simulink model "mono_kanal"  (R2024a)
settings: Solver=VariableStepAuto  StartTime=0.0  StopTime=1122.0  RelTol=1e-5  AbsTol=1e-6
libraries: simulink x13, matrix_library x3, sharedutil x2, aerolibutil x1
settings Model: Creator=evgenijkondratev  LastModifiedBy=evgenijkondratev

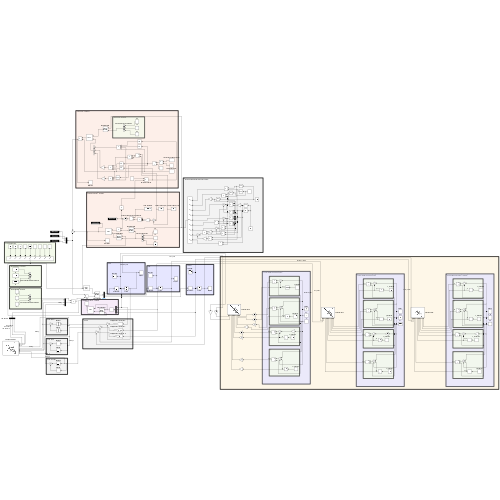
[thumbnail: Simulink's stored preview of the top-level diagram]
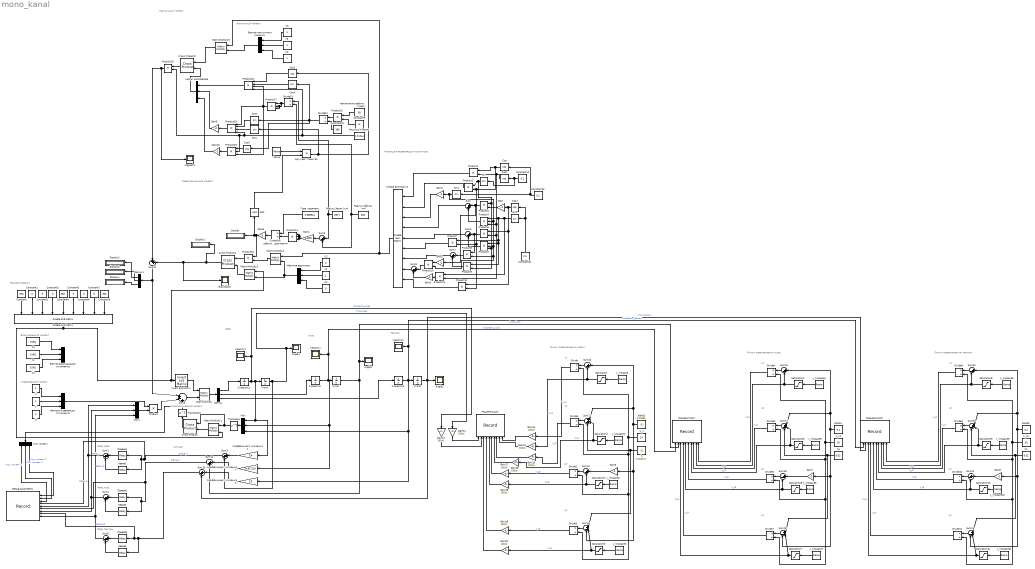
== system mono_kanal ==
  note: L3
  note: L2
  note: Тангаж
  note: L3
  note: L1
  note: Линии переключения (тангаж)
  note: L4
  note: L1
  note: Линии переключения (курс)
  note: Магнитный момент
  note: Реле, курс
  note: L4
  note: L3
  note: L4
  note: Сигнал
  note: L2
  note: Тензор инерции
  note: L2
  note: Реле, тангаж
  note: Магнитный момент
  note: Возмущающий момент
  note: Управляющий момент
  note: Крен
  note: Курс
  note: Реле, крен
  note: Матрица направляющих косинусов
  note: Гироскопический момент
  note: Гравитационный момент
  note: L1
  note: Линии переключения (крен)
  AngleX : Scope
  AngleY : Scope
  AngleZ : Scope
  Constant : Constant  Value=200
  Constant{1..3,5..7} (6 alike) : Constant  Value=0
  Constant10 : Constant  Value=180
  Constant11 : Constant  Value=0.1
  Constant12 : Constant  Value=0.1
  Constant13 : Constant  Value=0.1
  Constant4 : Constant  Value=250
  Constant8 : Constant  Value=300
  Constant9 : Constant  Value=pi
  Cos{,1..3,5} (5 alike) : Trigonometry  Operator=cos
  Cos4 : Trigonometry
  Create 3x3 Matrix : sharedutil/Create 3x3 Matrix  aMode=aMode
      settings: LibrarySourceBlock=aerolibutil/Create 3x3 Matrix
  Create 3x3 Matrix1 : sharedutil/Create 3x3 Matrix  aMode=aMode
      settings: LibrarySourceBlock=aerolibutil/Create 3x3 Matrix
  Cross Product : matrix_library/Cross Product
  Cross Product1 : matrix_library/Cross Product
  Cross Product2 : matrix_library/Cross Product
  Debug parameters : Record  FileSettingsInternal="{\"entries\":[{\"content\":{\"excelSettings\":{\"content\":{},\"type\":\"Streamout.ExcelSettings\"}},\"type\":\"Streamout.FileSettingStorage\",\"uuid\":\"\"}],\"packageUris\":[\"http:\\/\\/schema.mathworks.com\\/mf0\\/streamout_blocks\\/R2020a\"],\"version\":\"1.0\"}"  Layout=[1 1]  SignalsInternal="{\"entries\":[{\"content\":{\"signals\":[{\"content\":{\"blockPath\":[],\"dimensions\":[1,1],\"domain\":\"\",\"lineColor\":\"#a2142f\",\"plots\":[ 1 ],\"port\":1,\"sid\":[\"\"],\"signalID\":1,\"signalName\":\"Гир. момент Z\"},\"type\":\"RecordBlkView.Signal\",\"uuid\":\"\"},{\"content\":{\"blockPath\":[],\"dimensions\":[1,1],\"domain\":\"\",\"lineColor\":\"#139fff\",\"plots\":[ 1 ],\"port\":2,\"sid\":[\"\"],\"signalID\":2,\"signalName\":\"Гир. момент Y\"},\"type\":\"RecordBlkView.Signal\",\"uuid\":\"\"},{\"content\":{\"blockPath\":[],\"dimensions\":[1,1],\"domain\":\"\",\"lineColor\":\"#64d413\",\"lineWidth\":2,\"port\":3,\"sid\":[\"\"],\"signalID\":3,\"signalName\":\"Гир. момент X\"},\"type\":\"RecordBlkView.Signal\",\"uuid\":\"\"},{\"content\":{\"blockPath\":[],\"dimensions\":[1],\"domain\":\"\",\"lineColor\":\"#ff13a6\",\"lineWidth\":2,\"port\":4,\"sid\":[\"\"],\"signalID\":4,\"signalName\":\"Sigma_X\"},\"type\":\"RecordBlkView.Signal\",\"uuid\":\"\"},{\"content\":{\"blockPath\":[],\"dimensions\":[1],\"domain\":\"\",\"lineColor\":\"#fe330a\",\"lineWidth\":2,\"port\":5,\"sid\":[\"\"],\"signalID\":5,\"signalName\":\"Relay_X\"},\"type\":\"RecordBlkView.Signal\",\"uuid\":\"\"},{\"content\":{\"blockPath\":[],\"dimensions\":[1],\"domain\":\"\",\"lineColor\":\"#22b573\",\"lineWidth\":2,\"port\":6,\"sid\":[\"\"],\"signalID\":6,\"signalName\":\"Sigma_Y\"},\"type\":\"RecordBlkView.Signal\",\"uuid\":\"\"},{\"content\":{\"blockPath\":[],\"dimensions\":[1],\"domain\":\"\",\"lineColor\":\"#0072bd\",\"lineWidth\":2,\"port\":7,\"sid\":[\"\"],\"signalID\":7,\"signalName\":\"Relay_Y\"},\"type\":\"RecordBlkView.Signal\",\"uuid\":\"\"},{\"content\":{\"blockPath\":[],\"dimensions\":[1],\"domain\":\"\",\"lineColor\":\"#d95319\",\"lineWidth\":2,\"port\":8,\"sid\":[\"\"],\"signalID\":8,\"signalName\":\"Sigma_Z\"},\"type\":\"RecordBlkView.Signal\",\"uuid\":\"\"},{\"content\":{\"blockPath\":[],\"dimensions\":[1],\"domain\":\"\",\"lineColor\":\"#edb120\",\"lineWidth\":2,\"port\":9,\"sid\":[\"\"],\"signalID\":9,\"signalName\":\"Relay_Z\"},\"type\":\"RecordBlkView.Signal\",\"uuid\":\"\"}]},\"type\":\"RecordBlkView.InputSignals\",\"uuid\":\"\"}],\"packageUris\":[\"http:\\/\\/schema.mathworks.com\\/mf0\\/streamout_blocks\\/R2020a\"],\"version\":\"1.0\"}"  VisualizationBindings="{\"xyplotplugin\":{\"info\":[{\"series\":[{\"bindingParametersList\":[{\"parameter\":\"X-Axis\",\"signalID\":1,\"signalName\":\"Гир. момент Z\"},{\"parameter\":\"Y-Axis\",\"signalID\":2,\"signalName\":\"Гир. момент Y\"}],\"seriesID\":0}],\"subplotID\":1}]}}"  CompatibilityTag=XY
  Demux : Demux  Outputs=3
  Demux1 : Demux  Outputs=3
  Display{,1..4} (5 alike) : Display
  Divide{,1..13} (14 alike) : Product  Inputs=*/
  Gain{,1..3,6..8,10} (8 alike) : Gain  Gain=-1
  Gain{11..20} (10 alike) : Gain  Gain=180/pi
  Gain4 : Gain  Gain=1000
  Gain5 : Gain  Gain=3
  Gain9 : Gain  Gain=-2
  Gravitation : Scope
  Invert 3x3 Matrix : aerolibutil/Invert  3x3 Matrix
  Magnetic : Scope
  MatrixMultiply{,1..3,5} (5 alike) : Product  Multiplication=Matrix(*)
  Mux : Mux  Inputs=3
  Mux1 : Mux  Inputs=3
  PhasePortraitX : Record  FileSettingsInternal="{\"entries\":[{\"content\":{\"excelSettings\":{\"content\":{},\"type\":\"Streamout.ExcelSettings\"}},\"type\":\"Streamout.FileSettingStorage\",\"uuid\":\"\"}],\"packageUris\":[\"http:\\/\\/schema.mathworks.com\\/mf0\\/streamout_blocks\\/R2020a\"],\"version\":\"1.0\"}"  Layout=[1 1]  SignalsInternal="{\"entries\":[{\"content\":{\"signals\":[{\"content\":{\"blockPath\":[],\"dimensions\":[1],\"domain\":\"\",\"lineColor\":\"#a2142f\",\"lineWidth\":2,\"port\":1,\"sid\":[\"\"],\"signalID\":1,\"signalName\":\"Gain11\"},\"type\":\"RecordBlkView.Signal\",\"uuid\":\"\"},{\"content\":{\"blockPath\":[],\"dimensions\":[1],\"domain\":\"\",\"lineColor\":\"#139fff\",\"lineWidth\":2,\"port\":2,\"sid\":[\"\"],\"signalID\":2,\"signalName\":\"Gain12\"},\"type\":\"RecordBlkView.Signal\",\"uuid\":\"\"},{\"content\":{\"blockPath\":[],\"dimensions\":[1],\"domain\":\"\",\"lineColor\":\"#ff6929\",\"lineWidth\":2,\"port\":3,\"sid\":[\"\"],\"signalID\":3,\"signalName\":\"Gain20\"},\"type\":\"RecordBlkView.Signal\",\"uuid\":\"\"},{\"content\":{\"blockPath\":[],\"dimensions\":[1],\"domain\":\"\",\"lineColor\":\"#b746ff\",\"lineWidth\":2,\"port\":4,\"sid\":[\"\"],\"signalID\":4,\"signalName\":\"Gain19\"},\"type\":\"RecordBlkView.Signal\",\"uuid\":\"\"},{\"content\":{\"blockPath\":[],\"dimensions\":[1],\"domain\":\"\",\"lineColor\":\"#64d413\",\"lineWidth\":2,\"port\":5,\"sid\":[\"\"],\"signalID\":5,\"signalName\":\"Gain18\"},\"type\":\"RecordBlkView.Signal\",\"uuid\":\"\"},{\"content\":{\"blockPath\":[],\"dimensions\":[1],\"domain\":\"\",\"lineColor\":\"#ff13a6\",\"lineWidth\":2,\"port\":6,\"sid\":[\"\"],\"signalID\":6,\"signalName\":\"Gain17\"},\"type\":\"RecordBlkView.Signal\",\"uuid\":\"\"},{\"content\":{\"blockPath\":[],\"dimensions\":[1],\"domain\":\"\",\"lineColor\":\"#fe330a\",\"lineWidth\":2,\"port\":7,\"sid\":[\"\"],\"signalID\":7,\"signalName\":\"Gain16\"},\"type\":\"RecordBlkView.Signal\",\"uuid\":\"\"},{\"content\":{\"blockPath\":[],\"dimensions\":[1],\"domain\":\"\",\"lineColor\":\"#22b573\",\"lineWidth\":2,\"port\":8,\"sid\":[\"\"],\"signalID\":8,\"signalName\":\"Gain15\"},\"type\":\"RecordBlkView.Signal\",\"uuid\":\"\"},{\"content\":{\"blockPath\":[],\"dimensions\":[1],\"domain\":\"\",\"lineColor\":\"#0072bd\",\"lineWidth\":2,\"port\":9,\"sid\":[\"\"],\"signalID\":9,\"signalName\":\"Gain14\"},\"type\":\"RecordBlkView.Signal\",\"uuid\":\"\"},{\"content\":{\"blockPath\":[],\"dimensions\":[1],\"domain\":\"\",\"lineColor\":\"#d95319\",\"lineWidth\":2,\"port\":10,\"sid\":[\"\"],\"signalID\":10,\"signalName\":\"Gain13\"},\"type\":\"RecordBlkView.Signal\",\"uuid\":\"\"}]},\"type\":\"RecordBlkView.InputSignals\",\"uuid\":\"\"}],\"packageUris\":[\"http:\\/\\/schema.mathworks.com\\/mf0\\/streamout_blocks\\/R2020a\"],\"version\":\"1.0\"}"  VisualizationBindings="{\"xyplotplugin\":{\"info\":[{\"series\":[],\"subplotID\":1}]}}"  CompatibilityTag=XY
  PhasePortraitY : Record  FileSettingsInternal="{\"entries\":[{\"content\":{\"excelSettings\":{\"content\":{},\"type\":\"Streamout.ExcelSettings\"}},\"type\":\"Streamout.FileSettingStorage\",\"uuid\":\"\"}],\"packageUris\":[\"http:\\/\\/schema.mathworks.com\\/mf0\\/streamout_blocks\\/R2020a\"],\"version\":\"1.0\"}"  Layout=[1 1]  SignalsInternal="{\"entries\":[{\"content\":{\"signals\":[{\"content\":{\"blockPath\":[],\"dimensions\":[1],\"domain\":\"\",\"lineColor\":\"#edb120\",\"lineWidth\":2,\"port\":1,\"sid\":[\"\"],\"signalID\":1,\"signalName\":\"Скорость_курс\"},\"type\":\"RecordBlkView.Signal\",\"uuid\":\"\"},{\"content\":{\"blockPath\":[],\"dimensions\":[1],\"domain\":\"\",\"lineColor\":\"#7e2f8e\",\"lineWidth\":2,\"port\":2,\"sid\":[\"\"],\"signalID\":2,\"signalName\":\"Угол_Курс\"},\"type\":\"RecordBlkView.Signal\",\"uuid\":\"\"},{\"content\":{\"blockPath\":[],\"dimensions\":[1],\"domain\":\"\",\"lineColor\":\"#77ac30\",\"lineWidth\":2,\"port\":3,\"sid\":[\"\"],\"signalID\":3,\"signalName\":\"X_L4\"},\"type\":\"RecordBlkView.Signal\",\"uuid\":\"\"},{\"content\":{\"blockPath\":[],\"dimensions\":[1],\"domain\":\"\",\"lineColor\":\"#4dbeee\",\"lineWidth\":2,\"port\":4,\"sid\":[\"\"],\"signalID\":4,\"signalName\":\"Y_L4\"},\"type\":\"RecordBlkView.Signal\",\"uuid\":\"\"},{\"content\":{\"blockPath\":[],\"dimensions\":[1],\"domain\":\"\",\"lineColor\":\"#a2142f\",\"lineWidth\":2,\"port\":5,\"sid\":[\"\"],\"signalID\":5,\"signalName\":\"X_L3\"},\"type\":\"RecordBlkView.Signal\",\"uuid\":\"\"},{\"content\":{\"blockPath\":[],\"dimensions\":[1],\"domain\":\"\",\"lineColor\":\"#139fff\",\"lineWidth\":2,\"port\":6,\"sid\":[\"\"],\"signalID\":6,\"signalName\":\"Y_L3\"},\"type\":\"RecordBlkView.Signal\",\"uuid\":\"\"},{\"content\":{\"blockPath\":[],\"dimensions\":[1],\"domain\":\"\",\"lineColor\":\"#ff6929\",\"lineWidth\":2,\"port\":7,\"sid\":[\"\"],\"signalID\":7,\"signalName\":\"X_L2\"},\"type\":\"RecordBlkView.Signal\",\"uuid\":\"\"},{\"content\":{\"blockPath\":[],\"dimensions\":[1],\"domain\":\"\",\"lineColor\":\"#b746ff\",\"lineWidth\":2,\"port\":8,\"sid\":[\"\"],\"signalID\":8,\"signalName\":\"Y_L2\"},\"type\":\"RecordBlkView.Signal\",\"uuid\":\"\"},{\"content\":{\"blockPath\":[],\"dimensions\":[1],\"domain\":\"\",\"lineColor\":\"#64d413\",\"lineWidth\":2,\"port\":9,\"sid\":[\"\"],\"signalID\":9,\"signalName\":\"X_L1\"},\"type\":\"RecordBlkView.Signal\",\"uuid\":\"\"},{\"content\":{\"blockPath\":[],\"dimensions\":[1],\"domain\":\"\",\"lineColor\":\"#ff13a6\",\"lineWidth\":2,\"port\":10,\"sid\":[\"\"],\"signalID\":10,\"signalName\":\"Y_L1\"},\"type\":\"RecordBlkView.Signal\",\"uuid\":\"\"}]},\"type\":\"RecordBlkView.InputSignals\",\"uuid\":\"\"}],\"packageUris\":[\"http:\\/\\/schema.mathworks.com\\/mf0\\/streamout_blocks\\/R2020a\"],\"version\":\"1.0\"}"  VisualizationBindings="{\"xyplotplugin\":{\"info\":[{\"series\":[],\"subplotID\":1}]}}"  CompatibilityTag=XY
  PhasePortraitZ : Record  FileSettingsInternal="{\"entries\":[{\"content\":{\"excelSettings\":{\"content\":{},\"type\":\"Streamout.ExcelSettings\"}},\"type\":\"Streamout.FileSettingStorage\",\"uuid\":\"\"}],\"packageUris\":[\"http:\\/\\/schema.mathworks.com\\/mf0\\/streamout_blocks\\/R2020a\"],\"version\":\"1.0\"}"  Layout=[1 1]  SignalsInternal="{\"entries\":[{\"content\":{\"signals\":[{\"content\":{\"blockPath\":[],\"dimensions\":[1],\"domain\":\"\",\"lineColor\":\"#fe330a\",\"plots\":[ 1 ],\"port\":1,\"sid\":[\"\"],\"signalID\":1,\"signalName\":\"Скорость_тангаж\"},\"type\":\"RecordBlkView.Signal\",\"uuid\":\"\"},{\"content\":{\"blockPath\":[],\"dimensions\":[1],\"domain\":\"\",\"lineColor\":\"#139fff\",\"plots\":[ 1 ],\"port\":2,\"sid\":[\"\"],\"signalID\":2,\"signalName\":\"Угол_тангаж\"},\"type\":\"RecordBlkView.Signal\",\"uuid\":\"\"},{\"content\":{\"blockPath\":[],\"dimensions\":[1],\"domain\":\"\",\"lineColor\":\"#fe330a\",\"lineWidth\":2,\"port\":3,\"sid\":[\"\"],\"signalID\":3,\"signalName\":\"X_L4\"},\"type\":\"RecordBlkView.Signal\",\"uuid\":\"\"},{\"content\":{\"blockPath\":[],\"dimensions\":[1],\"domain\":\"\",\"lineColor\":\"#22b573\",\"lineWidth\":2,\"port\":4,\"sid\":[\"\"],\"signalID\":4,\"signalName\":\"Y_L4\"},\"type\":\"RecordBlkView.Signal\",\"uuid\":\"\"},{\"content\":{\"blockPath\":[],\"dimensions\":[1],\"domain\":\"\",\"lineColor\":\"#0072bd\",\"lineWidth\":2,\"port\":5,\"sid\":[\"\"],\"signalID\":5,\"signalName\":\"X_L3\"},\"type\":\"RecordBlkView.Signal\",\"uuid\":\"\"},{\"content\":{\"blockPath\":[],\"dimensions\":[1],\"domain\":\"\",\"lineColor\":\"#d95319\",\"lineWidth\":2,\"port\":6,\"sid\":[\"\"],\"signalID\":6,\"signalName\":\"Y_L3\"},\"type\":\"RecordBlkView.Signal\",\"uuid\":\"\"},{\"content\":{\"blockPath\":[],\"dimensions\":[1],\"domain\":\"\",\"lineColor\":\"#edb120\",\"lineWidth\":2,\"port\":7,\"sid\":[\"\"],\"signalID\":7,\"signalName\":\"X_L2\"},\"type\":\"RecordBlkView.Signal\",\"uuid\":\"\"},{\"content\":{\"blockPath\":[],\"dimensions\":[1],\"domain\":\"\",\"lineColor\":\"#7e2f8e\",\"lineWidth\":2,\"port\":8,\"sid\":[\"\"],\"signalID\":8,\"signalName\":\"Y_L2\"},\"type\":\"RecordBlkView.Signal\",\"uuid\":\"\"},{\"content\":{\"blockPath\":[],\"dimensions\":[1],\"domain\":\"\",\"lineColor\":\"#77ac30\",\"lineWidth\":2,\"port\":9,\"sid\":[\"\"],\"signalID\":9,\"signalName\":\"X_L1\"},\"type\":\"RecordBlkView.Signal\",\"uuid\":\"\"},{\"content\":{\"blockPath\":[],\"dimensions\":[1],\"domain\":\"\",\"lineColor\":\"#4dbeee\",\"lineWidth\":2,\"port\":10,\"sid\":[\"\"],\"signalID\":10,\"signalName\":\"Y_L1\"},\"type\":\"RecordBlkView.Signal\",\"uuid\":\"\"}]},\"type\":\"RecordBlkView.InputSignals\",\"uuid\":\"\"}],\"packageUris\":[\"http:\\/\\/schema.mathworks.com\\/mf0\\/streamout_blocks\\/R2020a\"],\"version\":\"1.0\"}"  VisualizationBindings="{\"xyplotplugin\":{\"info\":[{\"series\":[{\"bindingParametersList\":[{\"parameter\":\"X-Axis\",\"signalID\":1,\"signalName\":\"Скорость_тангаж\"},{\"parameter\":\"Y-Axis\",\"signalID\":2,\"signalName\":\"Угол_тангаж\"}],\"seriesID\":0}],\"subplotID\":1}]}}"  CompatibilityTag=XY
  Product{,1..3,5,7..13,15,20} (14 alike) : Product
  Product{4,6,14,17,19} (5 alike) : Product  Inputs=3
  Product16 : Product  Inputs=4
  Product18 : Product  Inputs=4
  Ramp : simulink/Sources/Ramp  slope=1  start=0  InitialOutput=0
  Saturation{,1..11} (12 alike) : Saturate  UpperLimit=0.15  LowerLimit=-0.15
  Sin{,1..4} (5 alike) : Trigonometry
  Sqrt : Sqrt
  Sum{,1,3..9,14..15,24} (12 alike) : Sum  Inputs=|++
  Sum{10,12,16,18,20,22} (6 alike) : Sum  Inputs=|+-
  Sum{11,13,17,19,21,23} (6 alike) : Sum  Inputs=|+--
  Sum2 : Sum  Inputs=|+-+
  Transpose : Math  Operator=transpose
  Transpose1 : Math  Operator=transpose
  Vector Concatenate : Concatenate  NumInputs=3
  VelocityX : Scope
  VelocityY : Scope
  VelocityZ : Scope
  X : Constant
  X1 : Constant  Value=0.001
  X2 : Constant  Value=0
  X3 : Constant
  Y : Constant
  Y1 : Constant  Value=0.001
  Y2 : Constant
  Y3 : Constant
  Z : Constant
  Z1 : Constant  Value=0.001
  Z2 : Constant  Value=0
  Z3 : Constant
  alpha1 : Constant  Value=0.1
  alpha2 : Constant  Value=0.00698
  alpha3 : Constant  Value=0.1
  h : Constant  Value=0.002617
  h1 : Constant  Value=0.02
  h2 : Constant  Value=0.02
  k_x : Constant  Value=14
  k_x1 : Constant  Value=10
  k_x2 : Constant  Value=10
  x_linspace{,1..11} (12 alike) : simulink/Sources/Ramp  slope=1  start=0  InitialOutput=-1
  Аргумент перигея : Product
  Вектор возмущающего момента : Concatenate  NumInputs=3
  Вектор магнитного момента : Concatenate  NumInputs=3
  Вектор управляющего момента : Concatenate  NumInputs=3
  Гир. момент : Demux  Outputs=3
  Грав. параметр : Constant  Value=3.986e14
  Индукция Земли : Constant  Value=0.315e-4
  Коэффициент усиления X : Gain  Gain=14
  Коэффициент усиления Y : Gain  Gain=14.617224
  Коэффициент усиления Z : Gain  Gain=10
  Левое1 : Relay  OnSwitchValue=-0.00698+0.002617  OffSwitchValue=-0.00698  OnOutputValue=0  OffOutputValue=-1
  Левое2 : Relay  OnSwitchValue=-0.08  OffSwitchValue=-0.1  OnOutputValue=0  OffOutputValue=-1
  Левое3 : Relay  OnSwitchValue=-0.08  OffSwitchValue=-0.1  OnOutputValue=0  OffOutputValue=-1
  Местная вертикаль : Concatenate  NumInputs=3
  Наклонение орбиты (град) : Constant  Value=50
  Правое1 : Relay  OnSwitchValue=0.00698  OffSwitchValue=0.00698-0.002617
  Правое2 : Relay  OnSwitchValue=0.1  OffSwitchValue=0.08
  Правое3 : Relay  OnSwitchValue=0.1  OffSwitchValue=0.08
  Радиус Земли (км) : Constant  Value=6371
  Радиус орбиты (км) : Constant  Value=820
  Скорость орбитального движения : Product  Inputs=*/
  СкоростьX : Integrator  InitialCondition=0.000114843
  СкоростьY : Integrator  InitialCondition=0.001
  СкоростьZ : Integrator  InitialCondition=0.001
  УголX : Integrator  InitialCondition=-0.0017558
  УголY : Integrator  InitialCondition=0.001
  УголZ : Integrator  InitialCondition=0.001
  wires:
  Gain1/1 -> Create 3x3 Matrix1/3
  Product3/1 -> Gain2/1, Sum/1
  Divide3/1 -> Gain19/1  "Y_L4"
  Sum22/1 -> Divide10/1
  Transpose1/1 -> Гир. момент/1
  Vector Concatenate/1 -> Cross Product2/2
  Sum6/1 -> Create 3x3 Matrix1/5
  Sum21/1 -> Divide9/1
  Sum13/1 -> Divide3/1
  Местная вертикаль/1 -> MatrixMultiply3/2, MatrixMultiply2/2
  Saturation4/1 -> PhasePortraitY/9, Sum16/2  "X_L1"
  Радиус орбиты (км)/1 -> Sum9/2, Divide13/2
  x_linspace2/1 -> Saturation2/1
  Sum11/1 -> Divide1/1
  УголY/1 -> PhasePortraitY/2, AngleY/1, Sum14/2  "Угол_Курс"
  x_linspace9/1 -> Saturation9/1
  Product6/1 -> Sum6/2
  X2/1 -> Местная вертикаль/1
  УголZ/1 -> PhasePortraitZ/2, Sum15/2, AngleZ/1  "Угол_тангаж"
  Gain4/1 -> Product14/1, Product14/2, Product14/3
  Gain2/1 -> Product10/1
  x_linspace8/1 -> Saturation8/1
  Sin/1 -> Product2/1, Product9/2, Product6/3, Product3/1
  Gain6/1 -> Sum12/1
  Divide10/1 -> PhasePortraitZ/6  "Y_L3"
  alpha1/1 -> Gain7/1, Sum19/3, Sum17/1, Sum16/1
  Sum15/1 -> Левое3/1, Debug parameters/8, Правое3/1  "Sigma_Z"
  Sum17/1 -> Divide5/1
  x_linspace10/1 -> Saturation10/1
  Z1/1 -> Вектор возмущающего момента/3
  Mux1/1 -> Product/2
  h1/1 -> Sum17/3, Sum19/1
  Product1/1 -> Create 3x3 Matrix1/1
  x_linspace1/1 -> Saturation1/1
  Product19/1 -> Gain10/1
  h2/1 -> Sum21/3, Sum23/1
  Ramp/1 -> Аргумент перигея/1
  Коэффициент усиления Y/1 -> Sum14/1
  Saturation7/1 -> PhasePortraitY/3, Sum19/2  "X_L4"
  Demux/3 -> СкоростьZ/1
  MatrixMultiply1/1 -> Cross Product/2
  Sum18/1 -> Divide6/1
  Sqrt/1 -> Аргумент перигея/2
  Sum12/1 -> Divide2/1
  Product4/1 -> Sum/2
  k_x/1 -> Divide3/2, Divide2/2, Divide1/2, Divide/2
  Sum8/1 -> Create 3x3 Matrix1/8
  Скорость орбитального движения/1 -> Gain5/1
  k_x2/1 -> Divide11/2, Divide10/2, Divide9/2, Divide8/2
  Cos1/1 -> Product1/2, Product11/2, Product5/2, Product4/3
  x_linspace11/1 -> Saturation11/1
  Product12/1 -> Create 3x3 Matrix1/9
  alpha3/1 -> Gain8/1, Sum23/3, Sum21/1, Sum20/1
  Product8/1 -> Sum7/1
  Saturation3/1 -> Gain20/1, Sum13/2  "X_L4"
  k_x1/1 -> Divide7/2, Divide6/2, Divide5/2, Divide4/2
  Вектор управляющего момента/1 -> Product/1
  Divide5/1 -> PhasePortraitY/8  "Y_L2"
  Sum4/1 -> Mux1/2, Debug parameters/7  "Relay_Y"
  Product14/1 -> Скорость орбитального движения/2
  Create 3x3 Matrix1/1 -> MatrixMultiply5/1, MatrixMultiply2/1
  MatrixMultiply5/1 -> Cross Product2/1
  Sum10/1 -> Divide/1
  Transpose/1 -> Cross Product/1, MatrixMultiply1/1
  x_linspace/1 -> Saturation/1
  Gain/1 -> Product3/2
  Create 3x3 Matrix/1 -> MatrixMultiply3/1, Invert 3x3 Matrix/1, MatrixMultiply1/2
  Invert 3x3 Matrix/1 -> MatrixMultiply/1
  MatrixMultiply/1 -> Demux/1
  Грав. параметр/1 -> Скорость орбитального движения/1
  Cross Product1/1 -> Display1/1, Sum24/2, Gravitation/1
  Product10/1 -> Sum8/1
  Sin2/1 -> Product11/1, Product6/1, Product9/1, Product7/1, Product4/1
  Product2/1 -> Create 3x3 Matrix1/2
  Cos3/1 -> Product16/1
  УголX/1 -> Gain11/1, AngleX/1, Sum3/2  "Угол_крен"
  h/1 -> Sum11/3, Sum13/1
  x_linspace7/1 -> Saturation7/1
  Product9/1 -> Sum7/2
  Saturation9/1 -> PhasePortraitZ/7, Sum21/2  "X_L2"
  Sum/1 -> Create 3x3 Matrix1/4
  Saturation2/1 -> Gain18/1, Sum12/2  "X_L3"
  Constant6/1 -> Create 3x3 Matrix/7
  Saturation1/1 -> Gain16/1, Sum11/2  "X_L2"
  Cos2/1 -> Product12/1, Product5/1, Gain/1
  Gain10/1 -> Vector Concatenate/3
  Z/1 -> Вектор управляющего момента/3
  X/1 -> Вектор управляющего момента/1
  Product18/1 -> Gain9/1
  Sum3/1 -> Debug parameters/4, Левое1/1, Правое1/1  "Sigma_X"
  X1/1 -> Вектор возмущающего момента/1
  Constant1/1 -> Create 3x3 Matrix/2
  Constant4/1 -> Create 3x3 Matrix/5
  Constant10/1 -> Divide12/2
  Gain7/1 -> Sum18/1
  Z2/1 -> Местная вертикаль/3
  Constant7/1 -> Create 3x3 Matrix/8
  Sum24/1 -> Sum2/1, Demux1/1
  Y1/1 -> Вектор возмущающего момента/2
  Sum2/1 -> MatrixMultiply/2
  Гир. момент/1 -> Debug parameters/3  "Гир. момент X"
  Product13/1 -> Cross Product1/1
  Product17/1 -> Product19/3, Product18/1, Product16/3
  Наклонение орбиты (град)/1 -> Product15/1
  Левое1/1 -> Sum1/2
  Saturation11/1 -> PhasePortraitZ/3, Sum23/2  "X_L4"
  СкоростьZ/1 -> PhasePortraitZ/1, VelocityZ/1, Коэффициент усиления Z/1, Mux/3, УголZ/1  "Скорость_тангаж"
  Y2/1 -> Местная вертикаль/2
  Правое3/1 -> Sum5/1
  Constant/1 -> Create 3x3 Matrix/1
  Product/1 -> Sum2/2
  Gain3/1 -> Sum8/2
  Sum1/1 -> Mux1/1, Debug parameters/5  "Relay_X"
  Sum5/1 -> Mux1/3, Debug parameters/9  "Relay_Z"
  Sum14/1 -> Левое2/1, Правое2/1, Debug parameters/6  "Sigma_Y"
  Product7/1 -> Create 3x3 Matrix1/6
  Constant2/1 -> Create 3x3 Matrix/3
  Demux/1 -> СкоростьX/1
  Гир. момент/2 -> Debug parameters/2  "Гир. момент Y"
  Cos/1 -> Product1/1, Product12/2, Product7/2, Product2/2
  Правое1/1 -> Sum1/1
  Индукция Земли/1 -> Product20/2, Product19/2, Product18/4, Product16/4
  Gain8/1 -> Sum22/1
  Product11/1 -> Gain3/1
  Product5/1 -> Product8/1, Sum6/1
  Gain9/1 -> Vector Concatenate/2
  x_linspace3/1 -> Saturation3/1
  Saturation6/1 -> PhasePortraitY/5, Sum18/2  "X_L3"
  Sum7/1 -> Create 3x3 Matrix1/7
  Divide9/1 -> PhasePortraitZ/8  "Y_L2"
  СкоростьY/1 -> VelocityY/1, PhasePortraitY/1, Mux/2, Коэффициент усиления Y/1, УголY/1  "Скорость_курс"
  Sin3/1 -> Product18/2
  Saturation/1 -> Gain14/1, Sum10/2  "X_L1"
  Divide6/1 -> PhasePortraitY/6  "Y_L3"
  Constant8/1 -> Create 3x3 Matrix/9
  Cos5/1 -> Product19/1
  Constant5/1 -> Create 3x3 Matrix/6
  Sum9/1 -> Gain4/1
  Sum23/1 -> Divide11/1
  Divide2/1 -> Gain17/1  "Y_L3"
  Cos4/1 -> Product16/2
  Demux/2 -> СкоростьY/1
  Product16/1 -> Vector Concatenate/1
  Divide1/1 -> Gain15/1  "Y_L2"
  Аргумент перигея/1 -> Sin4/1, Cos3/1
  Гир. момент/3 -> Debug parameters/1  "Гир. момент Z"
  Правое2/1 -> Sum4/1
  Gain5/1 -> Display/1, Sqrt/1, Product13/1
  Divide11/1 -> PhasePortraitZ/4  "Y_L4"
  Cross Product/1 -> Transpose1/1
  Y/1 -> Вектор управляющего момента/2
  Радиус Земли (км)/1 -> Divide13/1, Sum9/1
  Constant9/1 -> Product15/2
  Saturation5/1 -> PhasePortraitY/7, Sum17/2  "X_L2"
  alpha2/1 -> Gain6/1, Sum13/3, Sum11/1, Sum10/1
  Saturation8/1 -> PhasePortraitZ/9, Sum20/2  "X_L1"
  Коэффициент усиления X/1 -> Sum3/1
  Y3/1 -> Вектор магнитного момента/2
  Коэффициент усиления Z/1 -> Sum15/1
  x_linspace5/1 -> Saturation5/1
  Product15/1 -> Divide12/1
  Sum16/1 -> Divide4/1
  Divide13/1 -> Product17/1, Product17/3, Product17/2
  x_linspace6/1 -> Saturation6/1
  Z3/1 -> Вектор магнитного момента/3
  x_linspace4/1 -> Saturation4/1
  Sin1/1 -> Product10/2, Product8/2, Product6/2, Product4/2, Gain1/1
  Divide12/1 -> Sin3/1, Cos4/1, Cos5/1
  MatrixMultiply2/1 -> Product13/2
  Sum19/1 -> Divide7/1
  Product20/1 -> Sum24/1, Magnetic/1
  Mux/1 -> Transpose/1
  Divide/1 -> Gain13/1  "Y_L1"
  Saturation10/1 -> PhasePortraitZ/5, Sum22/2  "X_L3"
  Cross Product2/1 -> Product20/1
  Divide8/1 -> PhasePortraitZ/10  "Y_L1"
  Левое2/1 -> Sum4/2
  MatrixMultiply3/1 -> Cross Product1/2
  Divide4/1 -> PhasePortraitY/10  "Y_L1"
  Sin4/1 -> Product18/3
  Divide7/1 -> PhasePortraitY/4  "Y_L4"
  Вектор магнитного момента/1 -> MatrixMultiply5/2
  Sum20/1 -> Divide8/1
  СкоростьX/1 -> VelocityX/1, Gain12/1, Mux/1, Коэффициент усиления X/1, УголX/1  "Скорость_крен"
  X3/1 -> Вектор магнитного момента/1
  Constant3/1 -> Create 3x3 Matrix/4
  Левое3/1 -> Sum5/2
  Constant11/1 -> Sin2/1, Cos2/1
  Constant12/1 -> Sin/1, Cos1/1
  Constant13/1 -> Cos/1, Sin1/1
  Gain11/1 -> PhasePortraitX/1
  Gain12/1 -> PhasePortraitX/2
  Gain13/1 -> PhasePortraitX/10
  Gain14/1 -> PhasePortraitX/9
  Gain15/1 -> PhasePortraitX/8
  Gain16/1 -> PhasePortraitX/7
  Gain17/1 -> PhasePortraitX/6
  Gain18/1 -> PhasePortraitX/5
  Gain19/1 -> PhasePortraitX/4
  Gain20/1 -> PhasePortraitX/3
  Demux1/1 -> Display2/1
  Demux1/2 -> Display3/1
  Demux1/3 -> Display4/1
